simulink model "mock2dev_in"  (R2017b)
settings: Solver=VariableStepAuto  StartTime=0.0  StopTime=10  RelTol=1e-3
undefined symbols (not defined in the file or in its folder): sigbuilder_block
libraries: lib_ed247 x1
settings Model: Creator=odufour  LastModifiedBy=odufour
settings DataIOCC: InspectSignalLogs=on  ReturnWorkspaceOutputs=on
settings CodeAppCC: StateflowObjectComments=on

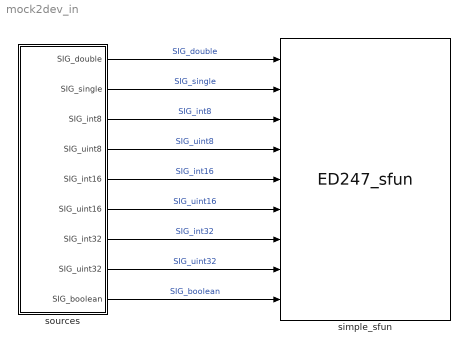
== system mock2dev_in ==
  simple_sfun : lib_ed247/ED247_sfun  configurationFilename='a429_uc_1_simple.xml'  enableLog=off  logFilename=''
      settings: SourceProductName=Airbus ED247
  sources : Subsystem  mask{Ts=2}
      mask prompts: Ts "Sample time"
  wires:
  sources/5(SIG_int16) -> simple_sfun/5  "SIG_int16"
  sources/2(SIG_single) -> simple_sfun/2  "SIG_single"
  sources/6(SIG_uint16) -> simple_sfun/6  "SIG_uint16"
  sources/7(SIG_int32) -> simple_sfun/7  "SIG_int32"
  sources/8(SIG_uint32) -> simple_sfun/8  "SIG_uint32"
  sources/3(SIG_int8) -> simple_sfun/3  "SIG_int8"
  sources/1(SIG_double) -> simple_sfun/1  "SIG_double"
  sources/9(SIG_boolean) -> simple_sfun/9  "SIG_boolean"
  sources/4(SIG_uint8) -> simple_sfun/4  "SIG_uint8"

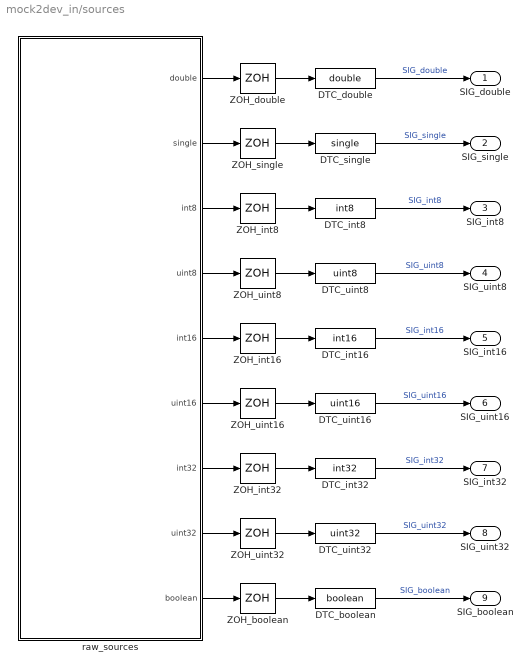
== system mock2dev_in/sources ==
  DTC_boolean : DataTypeConversion  OutDataTypeStr=boolean
  DTC_double : DataTypeConversion  OutDataTypeStr=double
  DTC_int16 : DataTypeConversion  OutDataTypeStr=int16
  DTC_int32 : DataTypeConversion  OutDataTypeStr=int32
  DTC_int8 : DataTypeConversion  OutDataTypeStr=int8
  DTC_single : DataTypeConversion  OutDataTypeStr=single
  DTC_uint16 : DataTypeConversion  OutDataTypeStr=uint16
  DTC_uint32 : DataTypeConversion  OutDataTypeStr=uint32
  DTC_uint8 : DataTypeConversion  OutDataTypeStr=uint8
  ZOH_boolean : ZeroOrderHold  SampleTime=Ts
  ZOH_double : ZeroOrderHold  SampleTime=Ts
  ZOH_int16 : ZeroOrderHold  SampleTime=Ts
  ZOH_int32 : ZeroOrderHold  SampleTime=Ts
  ZOH_int8 : ZeroOrderHold  SampleTime=Ts
  ZOH_single : ZeroOrderHold  SampleTime=Ts
  ZOH_uint16 : ZeroOrderHold  SampleTime=Ts
  ZOH_uint32 : ZeroOrderHold  SampleTime=Ts
  ZOH_uint8 : ZeroOrderHold  SampleTime=Ts
  raw_sources : Subsystem  Tag=STV Subsys  LoadFcn=sigbuilder_block('load');  StartFcn=sigbuilder_block('start');  StopFcn=sigbuilder_block('stop');  ClipboardFcn=sigbuilder_block('clipboard');  mask(Sigbuilder block){tuvar=[0:10]}
      mask help: Simulink:masks:SigbuilderBlock_MD
      mask init:
      | if ~strcmp(get_param(bdroot(gcbh),'SimulationStatus'),'stopped') tuvar = sigbuilder_block('maskInit'); end
      settings: CopyFcn=sigbuilder_block('copy');  DeleteFcn=sigbuilder_block('delete');  ModelCloseFcn=sigbuilder_block('modelClose');  PreSaveFcn=sigbuilder_block('preSave');  PauseFcn=sigbuilder_block('pause');  ContinueFcn=sigbuilder_block('continue');  NameChangeFcn=sigbuilder_block('namechange');  OpenFcn=sigbuilder_block('open',[6 22.5 1908 959.25 ]);  CloseFcn=sigbuilder_block('close');
      mask Display: plot(0, 0, 100, 100,[2, 2, 32, 32, 2], [68, 8, 8, 68, 68],[32, 2], [38, 38], [32, 19, 2],[53, 60, 44], [32, 17, 17, 2],[16, 16, 31, 31]);txt = getActiveGroup(gcbh);text(2, 100, txt,'verticalAlignment', 'top');
  SIG_double : Outport
  SIG_single : Outport  Port=2
  SIG_int8 : Outport  Port=3
  SIG_uint8 : Outport  Port=4
  SIG_int16 : Outport  Port=5
  SIG_uint16 : Outport  Port=6
  SIG_int32 : Outport  Port=7
  SIG_uint32 : Outport  Port=8
  SIG_boolean : Outport  Port=9
  wires:
  ZOH_int32/1 -> DTC_int32/1
  DTC_double/1 -> SIG_double/1  "SIG_double"
  ZOH_boolean/1 -> DTC_boolean/1
  ZOH_single/1 -> DTC_single/1
  ZOH_int8/1 -> DTC_int8/1
  ZOH_uint32/1 -> DTC_uint32/1
  ZOH_int16/1 -> DTC_int16/1
  ZOH_uint8/1 -> DTC_uint8/1
  DTC_uint16/1 -> SIG_uint16/1  "SIG_uint16"
  DTC_boolean/1 -> SIG_boolean/1  "SIG_boolean"
  DTC_single/1 -> SIG_single/1  "SIG_single"
  DTC_uint8/1 -> SIG_uint8/1  "SIG_uint8"
  DTC_int8/1 -> SIG_int8/1  "SIG_int8"
  DTC_int16/1 -> SIG_int16/1  "SIG_int16"
  DTC_int32/1 -> SIG_int32/1  "SIG_int32"
  DTC_uint32/1 -> SIG_uint32/1  "SIG_uint32"
  ZOH_uint16/1 -> DTC_uint16/1
  ZOH_double/1 -> DTC_double/1
  raw_sources/1(double) -> ZOH_double/1
  raw_sources/2(single) -> ZOH_single/1
  raw_sources/3(int8) -> ZOH_int8/1
  raw_sources/4(uint8) -> ZOH_uint8/1
  raw_sources/5(int16) -> ZOH_int16/1
  raw_sources/6(uint16) -> ZOH_uint16/1
  raw_sources/7(int32) -> ZOH_int32/1
  raw_sources/8(uint32) -> ZOH_uint32/1
  raw_sources/9(boolean) -> ZOH_boolean/1

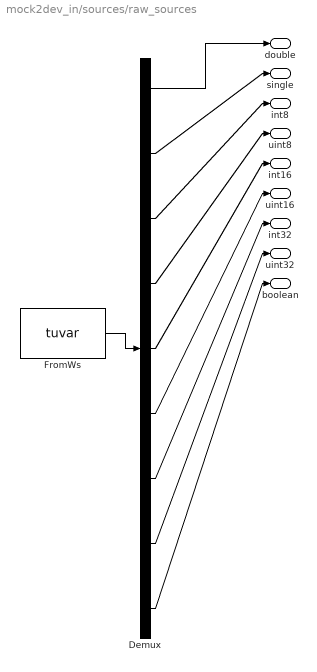
== system mock2dev_in/sources/raw_sources ==
  Demux : Demux  Tag=STV Demux  Outputs=9
  FromWs : FromWorkspace  Tag=STV FromWs  VariableName=tuvar  SampleTime=0
      SigBuilderData=|
      | common.afterFinalStr = 'Extrapolate'
      | common.sampleTime = 0
      | dataSet(1).timeRange = [0 10]
      | dataSet(1).name = 'Default'
      | dataSet(2).timeRange = [0 10]
      | dataSet(2).name = 'Constants'
      | sbobj.Groups(1).Name = 'Default'
      | sbobj.Groups(1).Signals(1).Name = 'double'
      | sbobj.Groups(1).Signals(1).XData = [0 4 4 6 6 10]
      | sbobj.Groups(1).Signals(1).YData = [0.5 0.5 1 1 42.3 42.3]
      | sbobj.Groups(1).Signals(2).Name = 'single'
      | sbobj.Groups(1).Signals(2).XData = [0 4 4 6 6 10]
      | sbobj.Groups(1).Signals(2).YData = [1.5 1.5 1 1 -6.4 -6.4]
      | sbobj.Groups(1).Signals(3).Name = 'int8'
      | sbobj.Groups(1).Signals(3).XData = [0 4 4 6 6 10]
      | sbobj.Groups(1).Signals(3).YData = [5 5 1 1 -102 -102]
      | sbobj.Groups(1).Signals(4).Name = 'uint8'
      | sbobj.Groups(1).Signals(4).XData = [0 4 4 6 6 10]
      | sbobj.Groups(1).Signals(4).YData = [4 4 1 1 205 205]
      | sbobj.Groups(1).Signals(5).Name = 'int16'
      | sbobj.Groups(1).Signals(5).XData = [0 4 4 6 6 10]
      | sbobj.Groups(1).Signals(5).YData = [-1250 -1250 1 1 987 987]
      | sbobj.Groups(1).Signals(6).Name = 'uint16'
      | sbobj.Groups(1).Signals(6).XData = [0 4 4 6 6 10]
      | sbobj.Groups(1).Signals(6).YData = [8 8 1 1 15 15]
      | sbobj.Groups(1).Signals(7).Name = 'int32'
      | sbobj.Groups(1).Signals(7).XData = [0 4 4 6 6 10]
      | sbobj.Groups(1).Signals(7).YData = [-5008 -5008 1 1 3009 3009]
      | sbobj.Groups(1).Signals(8).Name = 'uint32'
      | sbobj.Groups(1).Signals(8).XData = [0 4 4 6 6 10]
      | sbobj.Groups(1).Signals(8).YData = [14 14 1 1 6532 6532]
      | sbobj.Groups(1).Signals(9).Name = 'boolean'
      | sbobj.Groups(1).Signals(9).XData = [0 4 4 6 6 10]
      | sbobj.Groups(1).Signals(9).YData = [0 0 1 1 0 0]
      | sbobj.Groups(2).Name = 'Constants'
      | sbobj.Groups(2).Signals(1).Name = 'double'
      | sbobj.Groups(2).Signals(1).XData = [0 10]
      | sbobj.Groups(2).Signals(1).YData = [120.5 120.5]
      | sbobj.Groups(2).Signals(2).Name = 'single'
      | sbobj.Groups(2).Signals(2).XData = [0 10]
      | sbobj.Groups(2).Signals(2).YData = [1.5 1.5]
      | sbobj.Groups(2).Signals(3).Name = 'int8'
      | sbobj.Groups(2).Signals(3).XData = [0 10]
      | sbobj.Groups(2).Signals(3).YData = [5 5]
      | sbobj.Groups(2).Signals(4).Name = 'uint8'
      | sbobj.Groups(2).Signals(4).XData = [0 10]
      | sbobj.Groups(2).Signals(4).YData = [4 4]
      | sbobj.Groups(2).Signals(5).Name = 'int16'
      | sbobj.Groups(2).Signals(5).XData = [0 10]
      | sbobj.Groups(2).Signals(5).YData = [-1250 -1250]
      | sbobj.Groups(2).Signals(6).Name = 'uint16'
      | sbobj.Groups(2).Signals(6).XData = [0 10]
      | sbobj.Groups(2).Signals(6).YData = [8 8]
      | sbobj.Groups(2).Signals(7).Name = 'int32'
      | sbobj.Groups(2).Signals(7).XData = [0 10]
      | sbobj.Groups(2).Signals(7).YData = [-5000 -5000]
      | sbobj.Groups(2).Signals(8).Name = 'uint32'
      | sbobj.Groups(2).Signals(8).XData = [0 10]
      | sbobj.Groups(2).Signals(8).YData = [14 14]
      | sbobj.Groups(2).Signals(9).Name = 'boolean'
      | sbobj.Groups(2).Signals(9).XData = [0 10]
      | sbobj.Groups(2).Signals(9).YData = [1 1]
  double : Outport  Tag=STV Outport
  single : Outport  Tag=STV Outport  Port=2
  int8 : Outport  Tag=STV Outport  Port=3
  uint8 : Outport  Tag=STV Outport  Port=4
  int16 : Outport  Tag=STV Outport  Port=5
  uint16 : Outport  Tag=STV Outport  Port=6
  int32 : Outport  Tag=STV Outport  Port=7
  uint32 : Outport  Tag=STV Outport  Port=8
  boolean : Outport  Tag=STV Outport  Port=9
  wires:
  Demux/1 -> double/1
  FromWs/1 -> Demux/1
  Demux/2 -> single/1
  Demux/3 -> int8/1
  Demux/4 -> uint8/1
  Demux/5 -> int16/1
  Demux/6 -> uint16/1
  Demux/7 -> int32/1
  Demux/8 -> uint32/1
  Demux/9 -> boolean/1
